simulink model "simu_red_atraso"  (R2020b)
settings: Solver=VariableStepAuto  StartTime=0.0  StopTime=100  MaxStep=1e-3  RelTol=1e-3
values from neighbouring files (symbols this model uses):
  K = 1/div    [compensador_atraso.m]
  p = 0.001    [compensador_atraso.m]
  z = razon*p    (= 0.01)    [compensador_atraso.m]
libraries: simulink x1
settings Model: Creator=cmparedes  LastModifiedBy=Acer

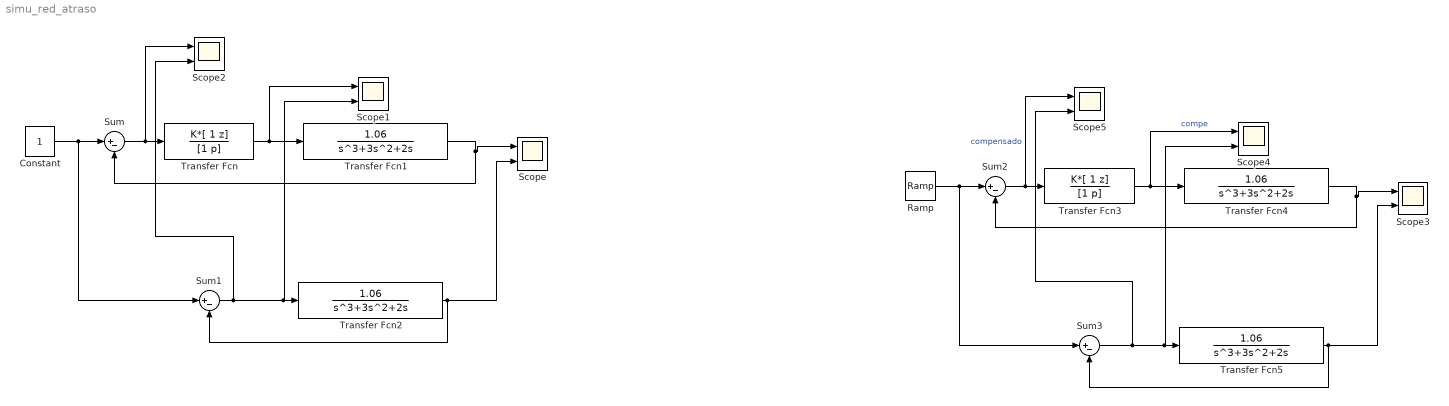
== system simu_red_atraso ==
  Constant : Constant
  Ramp : simulink/Sources/Ramp  slope=1  start=0  InitialOutput=0
  Scope{,1..5} (6 alike) : Scope  NumInputPorts=2
  Sum{,1..3} (4 alike) : Sum  Inputs=|+-
  Transfer Fcn : TransferFcn  Numerator=K*[ 1 z]  Denominator=[1 p]
  Transfer Fcn{1..2,4..5} (4 alike) : TransferFcn  Numerator=[1.06]  Denominator=[1 3 2 0]
  Transfer Fcn3 : TransferFcn  Numerator=K*[ 1 z]  Denominator=[1 p]
  wires:
  Sum/1 -> Scope2/1, Transfer Fcn/1
  Transfer Fcn/1 -> Scope1/1, Transfer Fcn1/1
  Transfer Fcn1/1 -> Sum/2, Scope/1
  Constant/1 -> Sum1/1, Sum/1
  Sum1/1 -> Scope2/2, Scope1/2, Transfer Fcn2/1
  Transfer Fcn2/1 -> Sum1/2, Scope/2
  Transfer Fcn5/1 -> Sum3/2, Scope3/2
  Transfer Fcn4/1 -> Sum2/2, Scope3/1
  Sum2/1 -> Scope5/1, Transfer Fcn3/1  "compensado"
  Sum3/1 -> Scope5/2, Scope4/2, Transfer Fcn5/1
  Transfer Fcn3/1 -> Scope4/1, Transfer Fcn4/1  "compe"
  Ramp/1 -> Sum3/1, Sum2/1
